simulink model "q5_descrete_adaptiv_controller"  (R2019a)
settings: Solver=VariableStepAuto  StartTime=0.0  StopTime=20  RelTol=1e-3
values from neighbouring files (symbols this model uses):
  dnum = hd.Denominator{1,1}    [adaptive_control_workspace.m]
  gama = 15    [adaptive_control_workspace.m]
  K = 10    [adaptive_control_workspace.m]
  k1 = 10    [adaptive_control_workspace.m]
  k2 = 10    [adaptive_control_workspace.m]
  lamda_0 = 7    [adaptive_control_workspace.m]
  m = 10    [adaptive_control_workspace.m]
  num = hd.Numerator{1,1}    [adaptive_control_workspace.m]
  TT = 0.05    [adaptive_control_workspace.m]
undefined symbols (not defined in the file or in its folder): DiscIntNeverNeededParam
libraries: simulink x3
settings Model: Creator=ronil  LastModifiedBy=ronil

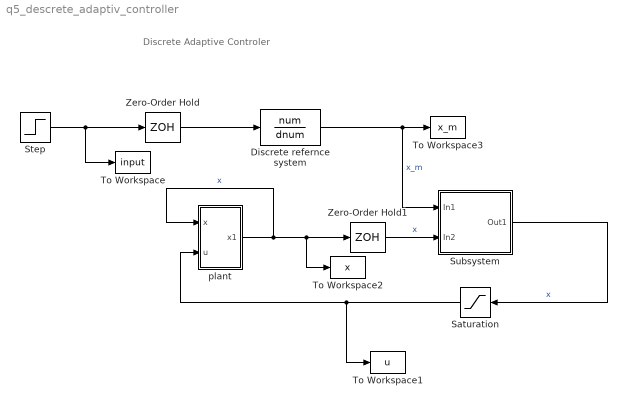
== system q5_descrete_adaptiv_controller ==
  note: Discrete Adaptive Controler
  Discrete refernce system : DiscreteTransferFcn  Numerator=num  Denominator=dnum
  Saturation : Saturate  UpperLimit=1000  LowerLimit=-1000
  Step : Step  SampleTime=0
  Subsystem : Subsystem
  To Workspace : ToWorkspace  VariableName=input  SaveFormat=Timeseries  SampleTime=-1
  To Workspace1 : ToWorkspace  VariableName=u  SaveFormat=Timeseries  SampleTime=-1
  To Workspace2 : ToWorkspace  VariableName=x  SaveFormat=Timeseries  SampleTime=-1
  To Workspace3 : ToWorkspace  VariableName=x_m  SaveFormat=Timeseries  SampleTime=-1
  Zero-Order Hold : ZeroOrderHold  SampleTime=TT
  Zero-Order Hold1 : ZeroOrderHold  SampleTime=TT
  plant : Subsystem
  wires:
  Step/1 -> To Workspace/1, Zero-Order Hold/1
  Discrete refernce system/1 -> To Workspace3/1, Subsystem/1(In1)  "x_m"
  plant/1(x1) -> plant/1(x), Zero-Order Hold1/1, To Workspace2/1  "x"
  Zero-Order Hold1/1 -> Subsystem/2(In2)  "x"
  Zero-Order Hold/1 -> Discrete refernce system/1
  Subsystem/1(Out1) -> Saturation/1  "x"
  Saturation/1 -> To Workspace1/1, plant/2(u)

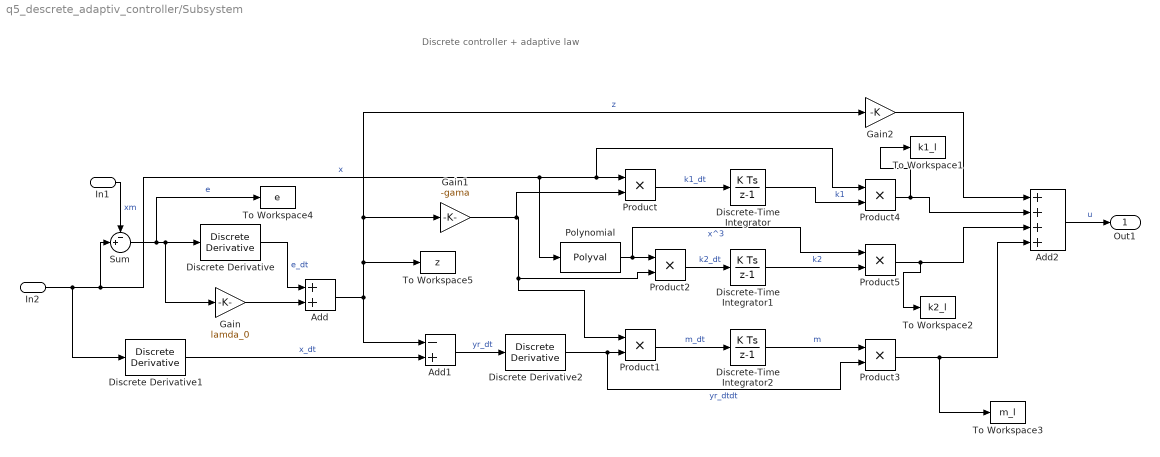
== system q5_descrete_adaptiv_controller/Subsystem ==
  note: Discrete controller + adaptive law
  In1 : Inport
  In2 : Inport  Port=2
  Add : Sum
  Add1 : Sum  Inputs=-+
  Add2 : Sum  Inputs=4
  Discrete Derivative : simulink/Discrete/Discrete Derivative  gainval=1.0  ICPrevScaledInput=0.0  OutMin=[]  OutMax=[]  OutDataType=fixdt(1, 16)  OutScaling=2^-10  DoSatur=off
  Discrete Derivative1 : simulink/Discrete/Discrete Derivative  gainval=1.0  ICPrevScaledInput=0.0  OutMin=[]  OutMax=[]  OutDataType=fixdt(1, 16)  OutScaling=2^-10  DoSatur=off
  Discrete Derivative2 : simulink/Discrete/Discrete Derivative  gainval=1.0  ICPrevScaledInput=0.0  OutMin=[]  OutMax=[]  OutDataType=fixdt(1, 16)  OutScaling=2^-10  DoSatur=off
  Discrete-Time Integrator : DiscreteIntegrator  SampleTime=-1  ICPrevOutput=DiscIntNeverNeededParam  ICPrevScaledInput=DiscIntNeverNeededParam
  Discrete-Time Integrator1 : DiscreteIntegrator  SampleTime=-1  ICPrevOutput=DiscIntNeverNeededParam  ICPrevScaledInput=DiscIntNeverNeededParam
  Discrete-Time Integrator2 : DiscreteIntegrator  SampleTime=-1  ICPrevOutput=DiscIntNeverNeededParam  ICPrevScaledInput=DiscIntNeverNeededParam
  Gain : Gain  Gain=lamda_0
  Gain1 : Gain  Gain=-gama
  Gain2 : Gain  Gain=-K
  Polynomial : Polyval  Coefs=[1 0 0 0]
  Product{,1..5} (6 alike) : Product
  Sum : Sum  Inputs=-+|
  To Workspace1 : ToWorkspace  VariableName=k1_l  SaveFormat=Timeseries  SampleTime=-1
  To Workspace2 : ToWorkspace  VariableName=k2_l  SaveFormat=Timeseries  SampleTime=-1
  To Workspace3 : ToWorkspace  VariableName=m_l  SaveFormat=Timeseries  SampleTime=-1
  To Workspace4 : ToWorkspace  VariableName=e  SaveFormat=Timeseries  SampleTime=-1
  To Workspace5 : ToWorkspace  VariableName=z  SaveFormat=Timeseries  SampleTime=-1
  Out1 : Outport  InitialOutput=[0]
  wires:
  In2/1 -> Product4/1, Product/1, Polynomial/1, Sum/2, Discrete Derivative1/1  "x"
  In1/1 -> Sum/1  "xm"
  Sum/1 -> To Workspace4/1, Discrete Derivative/1, Gain/1  "e"
  Add2/1 -> Out1/1  "u"
  Discrete Derivative/1 -> Add/1  "e_dt"
  Gain/1 -> Add/2
  Add/1 -> Add1/1, To Workspace5/1, Gain2/1, Gain1/1  "z"
  Discrete Derivative1/1 -> Add1/2  "x_dt"
  Add1/1 -> Discrete Derivative2/1  "yr_dt"
  Discrete Derivative2/1 -> Product3/2, Product1/2  "yr_dtdt"
  Gain1/1 -> Product/2, Product1/1, Product2/2
  Product1/1 -> Discrete-Time Integrator2/1  "m_dt"
  Polynomial/1 -> Product5/1, Product2/1  "x^3"
  Product2/1 -> Discrete-Time Integrator1/1  "k2_dt"
  Product/1 -> Discrete-Time Integrator/1  "k1_dt"
  Discrete-Time Integrator/1 -> Product4/2  "k1"
  Discrete-Time Integrator1/1 -> Product5/2  "k2"
  Discrete-Time Integrator2/1 -> Product3/1  "m"
  Gain2/1 -> Add2/1
  Product4/1 -> To Workspace1/1, Add2/2
  Product5/1 -> To Workspace2/1, Add2/3
  Product3/1 -> To Workspace3/1, Add2/4

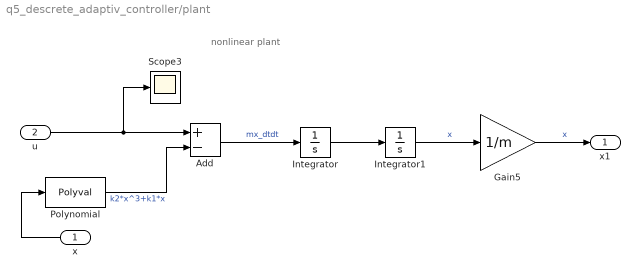
== system q5_descrete_adaptiv_controller/plant ==
  note: nonlinear plant
  x : Inport
  u : Inport  Port=2
  Add : Sum  Inputs=+-
  Gain5 : Gain  Gain=1/m
  Integrator : Integrator
  Integrator1 : Integrator
  Polynomial : Polyval  Coefs=[k2 0 k1 0]
  Scope3 : Scope
  x1 : Outport
  wires:
  Integrator/1 -> Integrator1/1
  Integrator1/1 -> Gain5/1  "x"
  Polynomial/1 -> Add/2  "k2*x^3+k1*x"
  x/1 -> Polynomial/1
  u/1 -> Add/1, Scope3/1
  Add/1 -> Integrator/1  "mx_dtdt"
  Gain5/1 -> x1/1  "x"
